simulink model "dist"  (R2025b)
settings: Solver=FixedStepDiscrete  StartTime=0.0  StopTime=inf  FixedStep=128/48000  RelTol=1e-3
model workspace (MATLAB code in the model file):
  | Gain_rt = Simulink.Parameter(1.0);
  | Bypass_rt = Simulink.Parameter(false);
undefined symbols (not defined in the file): Amount_rt, Asym_rt, Attack_rt, Level_rt, Mix_rt, Release_rt, Shaper_rt, Tone_rt
settings Model: Creator=linogarciamorales  LastModifiedBy=linogarciamorales
settings OptimizationCC: EnhancedBackFolding=on  PassReuseOutputArgsAs=Individual arguments  ZeroExternalMemoryAtStartup=off  ZeroInternalMemoryAtStartup=off  OptimizeBlockOrder=speed  DifferentSizesBufferReuse=on  OptimizationCustomize=off  EfficientTunableParamExpr=on
settings DebuggingCC: ParameterTunabilityLossMsg=error
settings SFSimCC: MATLABDynamicMemAlloc=off
settings RTWCC: SystemTargetFile=ert.tlc  GenCodeOnly=on  TemplateMakefile=ert_default_tmf  Description=Embedded Coder
settings CodeAppCC: ForceParamTrailComments=on  IgnoreCustomStorageClasses=off  OperatorAnnotations=on  SimulinkDataObjDesc=on  SFDataObjDesc=on  InsertBlockDesc=on
settings ERTTargetCC: InlinedParameterPlacement=Hierarchical  ERTCustomFileTemplate=example_file_process.tlc  TargetLangStandard=C99 (ISO)  GenerateSampleERTMain=on  SupportNonInlinedSFcns=on

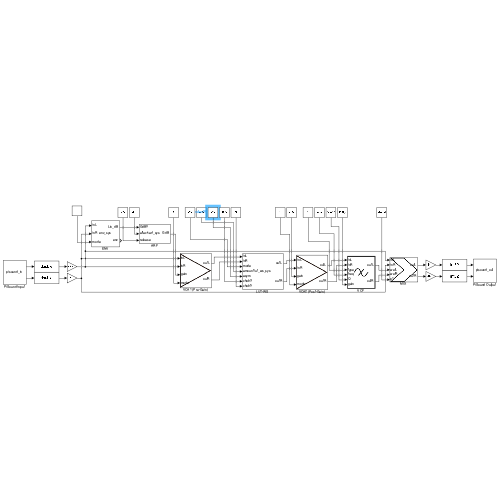
[thumbnail: Simulink's stored preview of the top-level diagram]
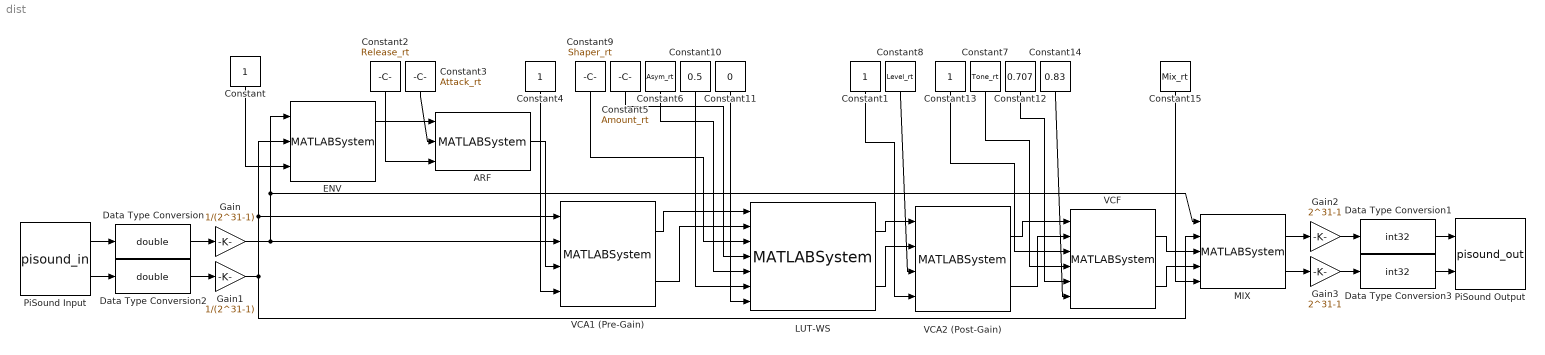
== system dist ==
  ARF : MATLABSystem  System=arf_sys  N=128  Fs=48000  AttackDefault=0.010  ReleaseDefault=0.100  SimulateUsing=Code generation
      mask Type: arf_sys
  Constant{,1,4,13} (4 alike) : Constant  OutDataTypeStr=uint8
  Constant10 : Constant  Value=0.5  OutDataTypeStr=double
  Constant11 : Constant  Value=0  OutDataTypeStr=double
  Constant12 : Constant  Value=0.707  OutDataTypeStr=double
  Constant14 : Constant  Value=0.83  OutDataTypeStr=double
  Constant15 : Constant  Value=Mix_rt  OutDataTypeStr=double
  Constant2 : Constant  Value=Release_rt  OutDataTypeStr=double
  Constant3 : Constant  Value=Attack_rt  OutDataTypeStr=double
  Constant5 : Constant  Value=Amount_rt  OutDataTypeStr=double
  Constant6 : Constant  Value=Asym_rt  OutDataTypeStr=double
  Constant7 : Constant  Value=Tone_rt  OutDataTypeStr=double
  Constant8 : Constant  Value=Level_rt  OutDataTypeStr=double
  Constant9 : Constant  Value=Shaper_rt  OutDataTypeStr=uint8
  Data Type Conversion : DataTypeConversion  OutDataTypeStr=double  SaturateOnIntegerOverflow=off  RndMeth=Floor
  Data Type Conversion1 : DataTypeConversion  OutDataTypeStr=int32  SaturateOnIntegerOverflow=off  RndMeth=Floor
  Data Type Conversion2 : DataTypeConversion  OutDataTypeStr=double  SaturateOnIntegerOverflow=off  RndMeth=Floor
  Data Type Conversion3 : DataTypeConversion  OutDataTypeStr=int32  SaturateOnIntegerOverflow=off  RndMeth=Floor
  ENV : MATLABSystem  System=env_sys  N=128  Fs=48000  ModeDefault=uint8( 1 )  Eps=1e-12  TauRMS=0.015  SimulateUsing=Code generation
      mask Type: env_sys
  Gain : Gain  Gain=1/(2^31-1)
  Gain1 : Gain  Gain=1/(2^31-1)
  Gain2 : Gain  Gain=2^31-1
  Gain3 : Gain  Gain=2^31-1
  LUT-WS : MATLABSystem  System=lut_ws_sys  N=128  M=257  bypass=uint8(0)  OS=uint8(1)  HB15=[ -1.06360599e-04, 0, 6.95210045e-03, 0, -5.16884606e-02, 0, 2.94825487e-01, 5.00034468e-01, 2.94825487e-01, 0, -5.16884606e-02, 0, 6.95210045e-03, 0, -1.06360599e-04 ]  ModeDefault=uint8( 3 )  AmountDefault=12.0  AsymDefault=0.0  Cheb3Default=1.0  Cheb5Default=0.0  XUser=linspace( -1, 1, 257 )  YUser=linspace( -1, 1, 257 )  MUser=257  Eps=1e-12  SimulateUsing=Code generation
      mask Type: lut_ws_sys
  MIX : MATLABSystem  System=mix_sys  N=128  Fs=48000  Mode=uint8( 0 )  SmoothTime=0.01  IndepInDB=false  SimulateUsing=Code generation
      mask Type: mix_sys
  PiSound Input : S-Function  FunctionName=pisound_in  Parameters=48000, 128, 0  SFunctionDeploymentMode=off  EnableBusSupport=off
  PiSound Output : S-Function  FunctionName=pisound_out  Parameters=48000, 128, 0  SFunctionDeploymentMode=off  EnableBusSupport=off
  VCA1 (Pre-Gain) : MATLABSystem  System=vca_sys  N=128  Fs=48000  bypass=uint8(0)  SimulateUsing=Code generation
      mask Type: vca_sys
  VCA2 (Post-Gain) : MATLABSystem  System=vca_sys  N=128  Fs=48000  bypass=uint8(0)  SimulateUsing=Code generation
      mask Type: vca_sys
  VCF : MATLABSystem  System=vcf_sys  N=128  Fs=48000  bypass=uint8(0)  SimulateUsing=Code generation
      mask Type: vcf_sys
  wires:
  PiSound Input/1 -> Data Type Conversion/1
  PiSound Input/2 -> Data Type Conversion2/1
  Data Type Conversion1/1 -> PiSound Output/1
  Data Type Conversion3/1 -> PiSound Output/2
  Gain2/1 -> Data Type Conversion1/1
  Gain3/1 -> Data Type Conversion3/1
  Data Type Conversion/1 -> Gain/1
  Data Type Conversion2/1 -> Gain1/1
  Gain/1 -> ENV/1, MIX/1, VCA1 (Pre-Gain)/2
  Gain1/1 -> MIX/2, ENV/2, VCA1 (Pre-Gain)/1
  Constant/1 -> ENV/3
  Constant1/1 -> VCA2 (Post-Gain)/4
  Constant2/1 -> ARF/3
  Constant3/1 -> ARF/2
  ARF/1 -> VCA1 (Pre-Gain)/3
  VCA1 (Pre-Gain)/1 -> LUT-WS/1
  VCA1 (Pre-Gain)/2 -> LUT-WS/2
  LUT-WS/1 -> VCA2 (Post-Gain)/1
  LUT-WS/2 -> VCA2 (Post-Gain)/2
  Constant8/1 -> VCA2 (Post-Gain)/3
  Constant9/1 -> LUT-WS/3
  Constant5/1 -> LUT-WS/4
  Constant6/1 -> LUT-WS/5
  Constant7/1 -> VCF/4
  VCA2 (Post-Gain)/1 -> VCF/1
  VCA2 (Post-Gain)/2 -> VCF/2
  ENV/1 -> ARF/1
  Constant4/1 -> VCA1 (Pre-Gain)/4
  Constant10/1 -> LUT-WS/6
  Constant11/1 -> LUT-WS/7
  Constant12/1 -> VCF/5
  Constant13/1 -> VCF/3
  Constant14/1 -> VCF/6
  MIX/1 -> Gain2/1
  MIX/2 -> Gain3/1
  VCF/1 -> MIX/3
  VCF/2 -> MIX/4
  Constant15/1 -> MIX/5
